simulink model "attitude_control_using_cots_rws_2ucubesat_final"  (R2019b)
settings: Solver=VariableStepAuto  StartTime=0.0  StopTime=5  RelTol=1e-3
libraries: dspmtrx3 x1, sharedutil x1, vrlib x1
settings Model: Creator=Asmaa  LastModifiedBy=AYSHA ALHARAM

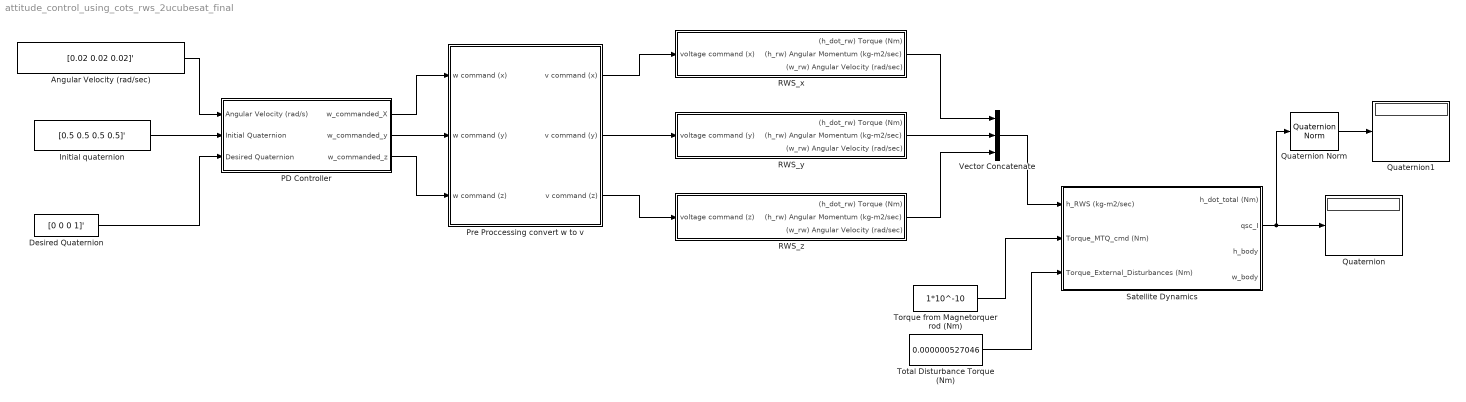
== system attitude_control_using_cots_rws_2ucubesat_final ==
  Angular Velocity (rad/sec) : Constant  Value=[0.02 0.02 0.02]'
  Desired Quaternion : Constant  Value=[0 0 0 1]'
  Initial quaternion : Constant  Value=[0.5 0.5 0.5 0.5]'
  PD Controller : Subsystem
  "Pre Proccessing convert w to v " : Subsystem
  Quaternion : Display
  Quaternion Norm : sharedutil/Quaternion Norm  aMode=aMode
      settings: SourceProductName=Aerospace Blockset  SourceProductBaseCode=AE
  Quaternion1 : Display
  "RWS_x " : Subsystem
  RWS_y : Subsystem
  RWS_z : Subsystem
  Satellite Dynamics : Subsystem
  Torque from Magnetorquer rod (Nm) : Constant  Value=1*10^-10
  Total Disturbance Torque (Nm) : Constant  Value=0.000000527046
  Vector Concatenate : Concatenate  NumInputs=3
  wires:
  "RWS_x "/2((h_rw) Angular Momentum (kg-m2/sec)) -> Vector Concatenate/1
  RWS_y/2((h_rw) Angular Momentum (kg-m2/sec)) -> Vector Concatenate/2
  RWS_z/2((h_rw) Angular Momentum (kg-m2/sec)) -> Vector Concatenate/3
  Vector Concatenate/1 -> Satellite Dynamics/1(h_RWS (kg-m2/sec))
  Total Disturbance Torque (Nm)/1 -> Satellite Dynamics/3(Torque_External_Disturbances (Nm))
  Satellite Dynamics/2(qsc_I) -> Quaternion/1, Quaternion Norm/1
  Initial quaternion/1 -> PD Controller/2(Initial Quaternion)
  PD Controller/1(w_commanded_X) -> "Pre Proccessing convert w to v "/1(w command (x))
  PD Controller/2(w_commanded_y) -> "Pre Proccessing convert w to v "/2(w command (y))
  PD Controller/3(w_commanded_z) -> "Pre Proccessing convert w to v "/3(w command (z))
  "Pre Proccessing convert w to v "/1(v command (x)) -> "RWS_x "/1(voltage command (x))
  "Pre Proccessing convert w to v "/2(v command (y)) -> RWS_y/1(voltage command (y))
  "Pre Proccessing convert w to v "/3(v command (z)) -> RWS_z/1(voltage command (z))
  Desired Quaternion/1 -> PD Controller/3(Desired Quaternion)
  Angular Velocity (rad/sec)/1 -> PD Controller/1(Angular Velocity (rad/s))
  Torque from Magnetorquer rod (Nm)/1 -> Satellite Dynamics/2(Torque_MTQ_cmd (Nm))
  Quaternion Norm/1 -> Quaternion1/1

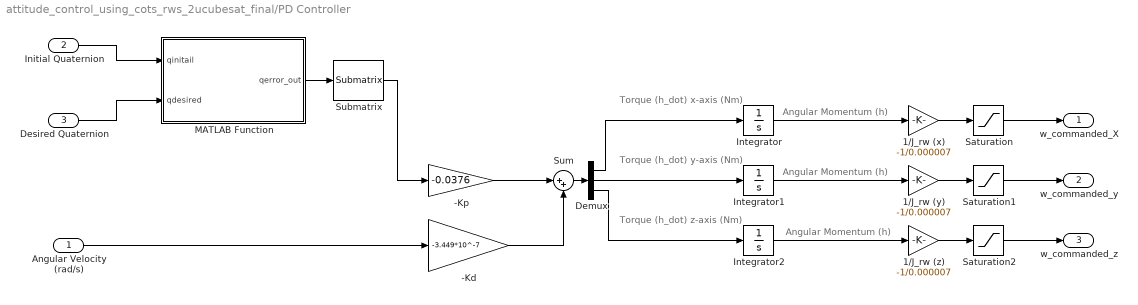
== system attitude_control_using_cots_rws_2ucubesat_final/PD Controller ==
  note: Angular Momentum (h)
  note: Torque (h_dot) x-axis (Nm)
  note: Torque (h_dot) y-axis (Nm)
  note: Torque (h_dot) z-axis (Nm)
  note: Angular Momentum (h)
  note: Angular Momentum (h)
  Angular Velocity (rad/s) : Inport
  Initial Quaternion : Inport  Port=2
  Desired Quaternion : Inport  Port=3
  -Kd : Gain  Gain=-3.449*10^-7
  -Kp : Gain  Gain=-0.0376
  1/J_rw (x) : Gain  Gain=-1/0.000007
  1/J_rw (y) : Gain  Gain=-1/0.000007
  1/J_rw (z) : Gain  Gain=-1/0.000007
  Demux : Demux  Outputs=3
  Integrator : Integrator
  Integrator1 : Integrator
  Integrator2 : Integrator
  MATLAB Function : MATLAB Function  TreatAsAtomicUnit=on
  Saturation : Saturate  UpperLimit=733.038285  LowerLimit=-733.038285  OutMin=-733.038286  OutMax=[733.038286]
  Saturation1 : Saturate  UpperLimit=733.038285  LowerLimit=-733.038285  OutMin=-733.038286  OutMax=[733.038286]
  Saturation2 : Saturate  UpperLimit=733.038285  LowerLimit=-733.038285  OutMin=-733.038286  OutMax=[733.038286]
  Submatrix : dspmtrx3/Submatrix  RowSpan=Range of rows  RowStartMode=Index  RowStartIndex=2  RowEndMode=Last  RowEndIndex=1  ColSpan=Range of columns  ColStartMode=First  ColStartIndex=1  ColEndMode=Last  ColEndIndex=1
  Sum : Sum  Inputs=|++
  w_commanded_X : Outport
  w_commanded_y : Outport  Port=2
  w_commanded_z : Outport  Port=3
  wires:
  Demux/3 -> Integrator2/1
  -Kd/1 -> Sum/2
  -Kp/1 -> Sum/1
  Sum/1 -> Demux/1
  Demux/2 -> Integrator1/1
  Integrator/1 -> 1/J_rw (x)/1
  Integrator1/1 -> 1/J_rw (y)/1
  Integrator2/1 -> 1/J_rw (z)/1
  Demux/1 -> Integrator/1
  1/J_rw (y)/1 -> Saturation1/1
  1/J_rw (z)/1 -> Saturation2/1
  Angular Velocity (rad/s)/1 -> -Kd/1
  1/J_rw (x)/1 -> Saturation/1
  Saturation/1 -> w_commanded_X/1
  Saturation1/1 -> w_commanded_y/1
  Saturation2/1 -> w_commanded_z/1
  Initial Quaternion/1 -> MATLAB Function/1(qinitail)
  Desired Quaternion/1 -> MATLAB Function/2(qdesired)
  MATLAB Function/1(qerror_out) -> Submatrix/1
  Submatrix/1 -> -Kp/1

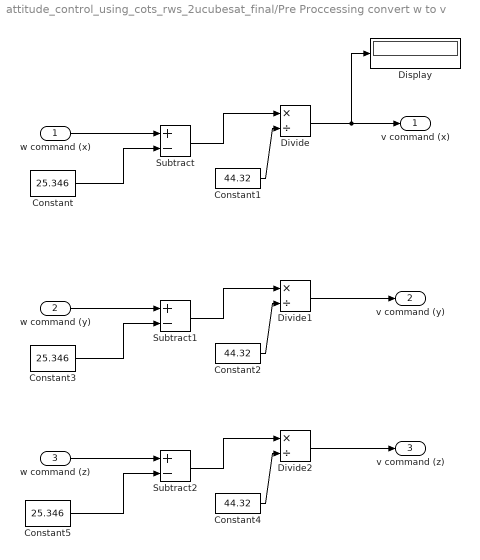
== system attitude_control_using_cots_rws_2ucubesat_final/Pre Proccessing convert w to v  ==
  w command (x) : Inport
  w command (y) : Inport  Port=2
  w command (z) : Inport  Port=3
  Constant : Constant  Value=25.346
  Constant1 : Constant  Value=44.32
  Constant2 : Constant  Value=44.32
  Constant3 : Constant  Value=25.346
  Constant4 : Constant  Value=44.32
  Constant5 : Constant  Value=25.346
  Display : Display
  Divide : Product  Inputs=*/
  Divide1 : Product  Inputs=*/
  Divide2 : Product  Inputs=*/
  Subtract : Sum  Inputs=+-
  Subtract1 : Sum  Inputs=+-
  Subtract2 : Sum  Inputs=+-
  v command (x) : Outport
  v command (y) : Outport  Port=2
  v command (z) : Outport  Port=3
  wires:
  w command (x)/1 -> Subtract/1
  Constant/1 -> Subtract/2
  Subtract/1 -> Divide/1
  Constant1/1 -> Divide/2
  Divide/1 -> Display/1, v command (x)/1
  Subtract1/1 -> Divide1/1
  Constant2/1 -> Divide1/2
  w command (y)/1 -> Subtract1/1
  Divide1/1 -> v command (y)/1
  Constant3/1 -> Subtract1/2
  w command (z)/1 -> Subtract2/1
  Constant4/1 -> Divide2/2
  Divide2/1 -> v command (z)/1
  Constant5/1 -> Subtract2/2
  Subtract2/1 -> Divide2/1

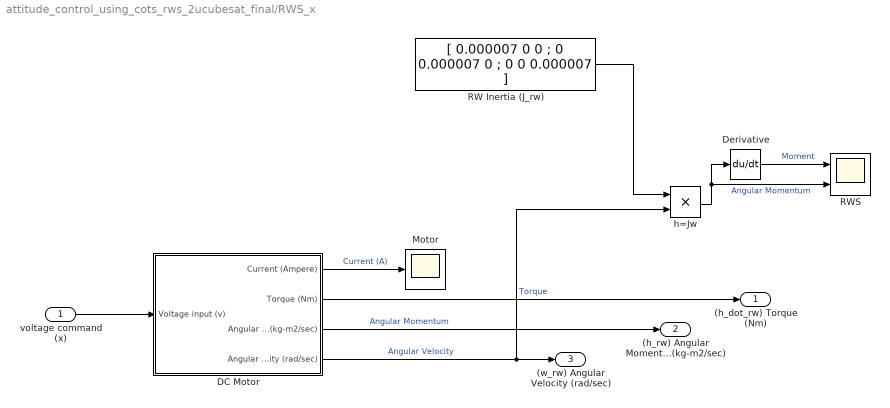
== system attitude_control_using_cots_rws_2ucubesat_final/RWS_x  ==
  voltage command (x) : Inport
  DC Motor : Subsystem
  Derivative : Derivative
  Motor : Scope
  RW Inertia (J_rw) : Constant  Value=[ 0.000007 0 0 ; 0 0.000007 0 ; 0 0 0.000007 ]
  RWS : Scope  NumInputPorts=2
  h=Jw : Product
  (h_dot_rw) Torque (Nm) : Outport
  (h_rw) Angular Momentum (kg-m2/sec) : Outport  Port=2
  (w_rw) Angular Velocity (rad/sec) : Outport  Port=3
  wires:
  RW Inertia (J_rw)/1 -> h=Jw/1
  DC Motor/2(Torque (Nm)) -> (h_dot_rw) Torque (Nm)/1  "Torque"
  h=Jw/1 -> Derivative/1, RWS/2  "Angular Momentum"
  voltage command (x)/1 -> DC Motor/1(Voltage input (v))
  Derivative/1 -> RWS/1  "Moment"
  DC Motor/4(Angular Velocity (rad/sec)) -> (w_rw) Angular Velocity (rad/sec)/1, h=Jw/2  "Angular Velocity"
  DC Motor/1(Current (Ampere)) -> Motor/1  "Current (A)"
  DC Motor/3(Angular Momentum (kg-m2/sec)) -> (h_rw) Angular Momentum (kg-m2/sec)/1  "Angular Momentum"

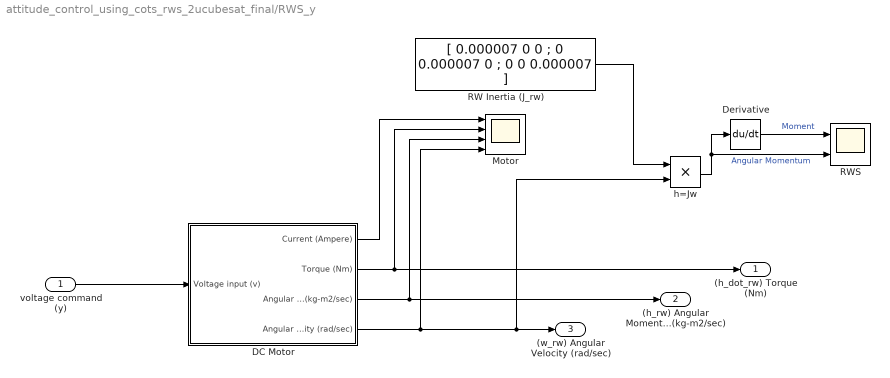
== system attitude_control_using_cots_rws_2ucubesat_final/RWS_y ==
  voltage command (y) : Inport
  DC Motor : Subsystem
  Derivative : Derivative
  Motor : Scope  NumInputPorts=4
  RW Inertia (J_rw) : Constant  Value=[ 0.000007 0 0 ; 0 0.000007 0 ; 0 0 0.000007 ]
  RWS : Scope  NumInputPorts=2
  h=Jw : Product
  (h_dot_rw) Torque (Nm) : Outport
  (h_rw) Angular Momentum (kg-m2/sec) : Outport  Port=2
  (w_rw) Angular Velocity (rad/sec) : Outport  Port=3
  wires:
  DC Motor/2(Torque (Nm)) -> (h_dot_rw) Torque (Nm)/1, Motor/2
  h=Jw/1 -> Derivative/1, RWS/2  "Angular Momentum"
  voltage command (y)/1 -> DC Motor/1(Voltage input (v))
  Derivative/1 -> RWS/1  "Moment"
  DC Motor/4(Angular Velocity (rad/sec)) -> Motor/4, (w_rw) Angular Velocity (rad/sec)/1, h=Jw/2
  DC Motor/1(Current (Ampere)) -> Motor/1
  DC Motor/3(Angular Momentum (kg-m2/sec)) -> (h_rw) Angular Momentum (kg-m2/sec)/1, Motor/3
  RW Inertia (J_rw)/1 -> h=Jw/1

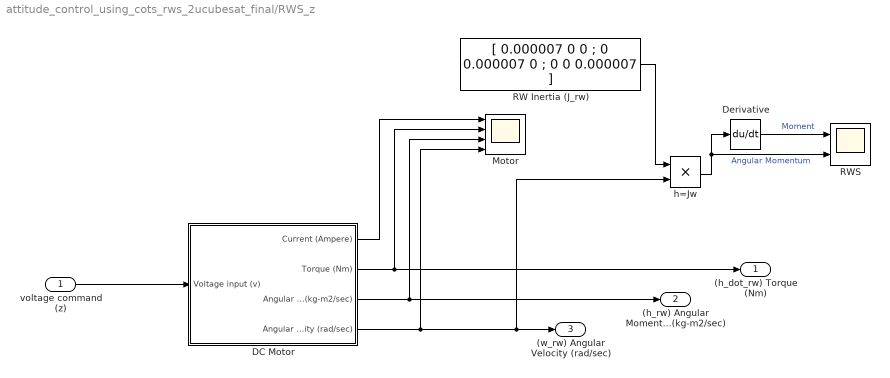
== system attitude_control_using_cots_rws_2ucubesat_final/RWS_z ==
  voltage command (z) : Inport
  DC Motor : Subsystem
  Derivative : Derivative
  Motor : Scope  NumInputPorts=4
  RW Inertia (J_rw) : Constant  Value=[ 0.000007 0 0 ; 0 0.000007 0 ; 0 0 0.000007 ]
  RWS : Scope  NumInputPorts=2
  h=Jw : Product
  (h_dot_rw) Torque (Nm) : Outport
  (h_rw) Angular Momentum (kg-m2/sec) : Outport  Port=2
  (w_rw) Angular Velocity (rad/sec) : Outport  Port=3
  wires:
  DC Motor/2(Torque (Nm)) -> (h_dot_rw) Torque (Nm)/1, Motor/2
  h=Jw/1 -> Derivative/1, RWS/2  "Angular Momentum"
  voltage command (z)/1 -> DC Motor/1(Voltage input (v))
  Derivative/1 -> RWS/1  "Moment"
  DC Motor/4(Angular Velocity (rad/sec)) -> Motor/4, (w_rw) Angular Velocity (rad/sec)/1, h=Jw/2
  DC Motor/1(Current (Ampere)) -> Motor/1
  DC Motor/3(Angular Momentum (kg-m2/sec)) -> (h_rw) Angular Momentum (kg-m2/sec)/1, Motor/3
  RW Inertia (J_rw)/1 -> h=Jw/1

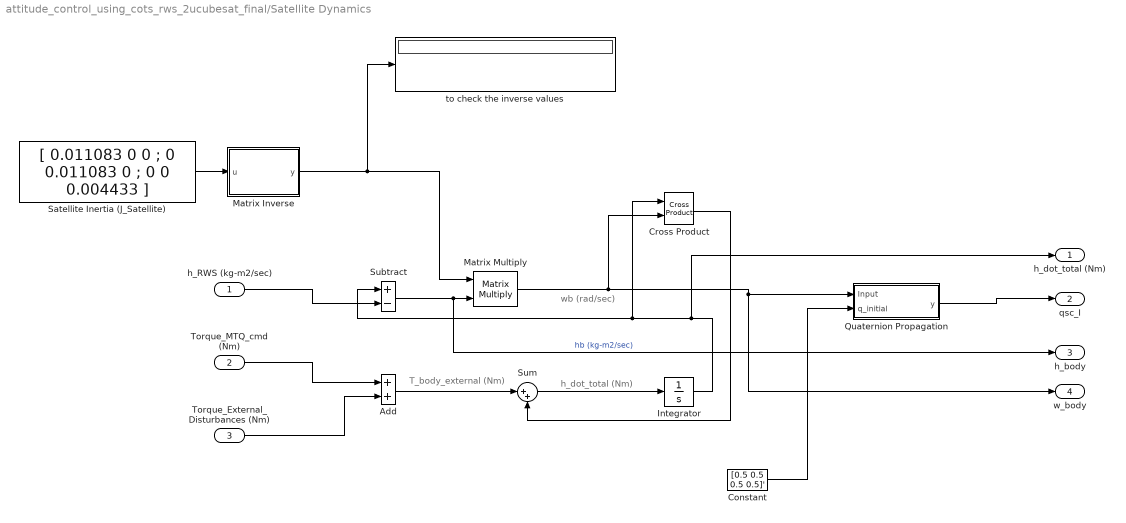
== system attitude_control_using_cots_rws_2ucubesat_final/Satellite Dynamics ==
  note: wb (rad/sec)
  note: T_body_external (Nm)
  note: h_dot_total (Nm)
  h_RWS (kg-m2/sec) : Inport
  Torque_MTQ_cmd (Nm) : Inport  Port=2
  Torque_External_Disturbances (Nm) : Inport  Port=3
  Add : Sum
  Constant : Constant  Value=[0.5 0.5 0.5 0.5]'
  Cross Product : vrlib/Utilities/Cross Product
  Integrator : Integrator
  Matrix Inverse : MATLAB Function  TreatAsAtomicUnit=on
  Matrix Multiply : Product  Multiplication=Matrix(*)
  "Quaternion Propagation " : Subsystem
  Satellite Inertia (J_Satellite) : Constant  Value=[ 0.011083 0 0 ; 0 0.011083 0 ; 0 0 0.004433 ]
  Subtract : Sum  Inputs=+-
  Sum : Sum  Inputs=|++
  to check the inverse values : Display
  h_dot_total (Nm) : Outport
  qsc_I : Outport  Port=2
  h_body : Outport  Port=3
  w_body : Outport  Port=4
  wires:
  Torque_MTQ_cmd (Nm)/1 -> Add/1
  Torque_External_Disturbances (Nm)/1 -> Add/2
  Add/1 -> Sum/1
  Sum/1 -> Integrator/1
  h_RWS (kg-m2/sec)/1 -> Subtract/2
  Subtract/1 -> h_body/1, Matrix Multiply/2  "hb (kg-m2/sec)"
  Matrix Inverse/1(y) -> to check the inverse values/1, Matrix Multiply/1
  Cross Product/1 -> Sum/2
  "Quaternion Propagation "/1(y) -> qsc_I/1
  Satellite Inertia (J_Satellite)/1 -> Matrix Inverse/1(u)
  Matrix Multiply/1 -> Cross Product/2, "Quaternion Propagation "/1(Input), w_body/1
  Integrator/1 -> h_dot_total (Nm)/1, Cross Product/1, Subtract/1
  Constant/1 -> "Quaternion Propagation "/2(q_initial)

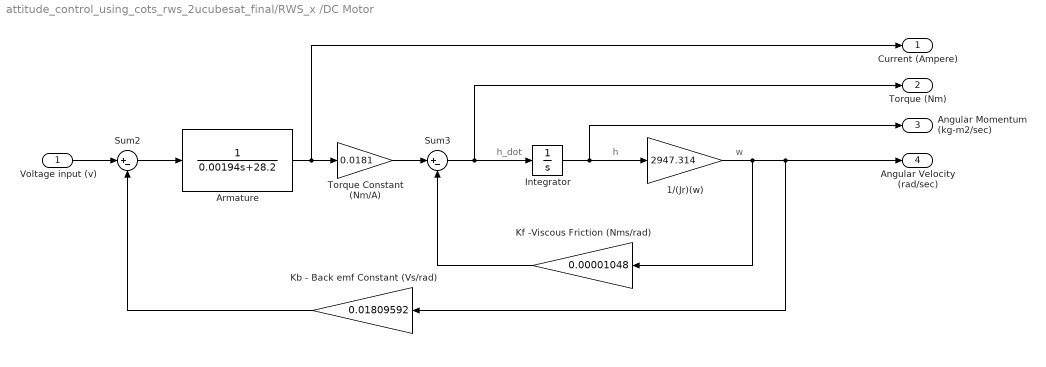
== system attitude_control_using_cots_rws_2ucubesat_final/RWS_x /DC Motor ==
  note: h_dot
  note: h
  note: w
  Voltage input (v) : Inport
  1/(Jr)(w) : Gain  Gain=2947.314
  Armature : TransferFcn  Denominator=[0.00194 28.2]
  Integrator : Integrator
  Kb - Back emf Constant (Vs/rad) : Gain  Gain=0.01809592
  Kf -Viscous Friction (Nms/rad) : Gain  Gain=0.00001048
  Sum2 : Sum  Inputs=|+-
  Sum3 : Sum  Inputs=|+-
  Torque Constant (Nm/A) : Gain  Gain=0.0181
  Current (Ampere) : Outport
  Torque (Nm) : Outport  Port=2
  Angular Momentum (kg-m2/sec) : Outport  Port=3
  Angular Velocity (rad/sec) : Outport  Port=4
  wires:
  Sum3/1 -> Integrator/1, Torque (Nm)/1
  Torque Constant (Nm/A)/1 -> Sum3/1
  Kb - Back emf Constant (Vs/rad)/1 -> Sum2/2
  Kf -Viscous Friction (Nms/rad)/1 -> Sum3/2
  Voltage input (v)/1 -> Sum2/1
  1/(Jr)(w)/1 -> Angular Velocity (rad/sec)/1, Kb - Back emf Constant (Vs/rad)/1, Kf -Viscous Friction (Nms/rad)/1
  Armature/1 -> Current (Ampere)/1, Torque Constant (Nm/A)/1
  Sum2/1 -> Armature/1
  Integrator/1 -> Angular Momentum (kg-m2/sec)/1, 1/(Jr)(w)/1

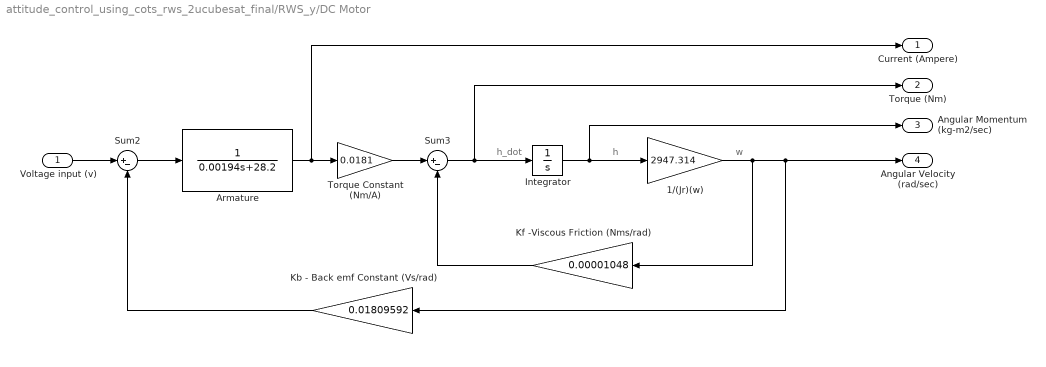
== system attitude_control_using_cots_rws_2ucubesat_final/RWS_y/DC Motor ==
  note: h_dot
  note: h
  note: w
  Voltage input (v) : Inport
  1/(Jr)(w) : Gain  Gain=2947.314
  Armature : TransferFcn  Denominator=[0.00194 28.2]
  Integrator : Integrator
  Kb - Back emf Constant (Vs/rad) : Gain  Gain=0.01809592
  Kf -Viscous Friction (Nms/rad) : Gain  Gain=0.00001048
  Sum2 : Sum  Inputs=|+-
  Sum3 : Sum  Inputs=|+-
  Torque Constant (Nm/A) : Gain  Gain=0.0181
  Current (Ampere) : Outport
  Torque (Nm) : Outport  Port=2
  Angular Momentum (kg-m2/sec) : Outport  Port=3
  Angular Velocity (rad/sec) : Outport  Port=4
  wires:
  Sum3/1 -> Integrator/1, Torque (Nm)/1
  Torque Constant (Nm/A)/1 -> Sum3/1
  Kb - Back emf Constant (Vs/rad)/1 -> Sum2/2
  Kf -Viscous Friction (Nms/rad)/1 -> Sum3/2
  Voltage input (v)/1 -> Sum2/1
  1/(Jr)(w)/1 -> Angular Velocity (rad/sec)/1, Kb - Back emf Constant (Vs/rad)/1, Kf -Viscous Friction (Nms/rad)/1
  Armature/1 -> Current (Ampere)/1, Torque Constant (Nm/A)/1
  Sum2/1 -> Armature/1
  Integrator/1 -> Angular Momentum (kg-m2/sec)/1, 1/(Jr)(w)/1

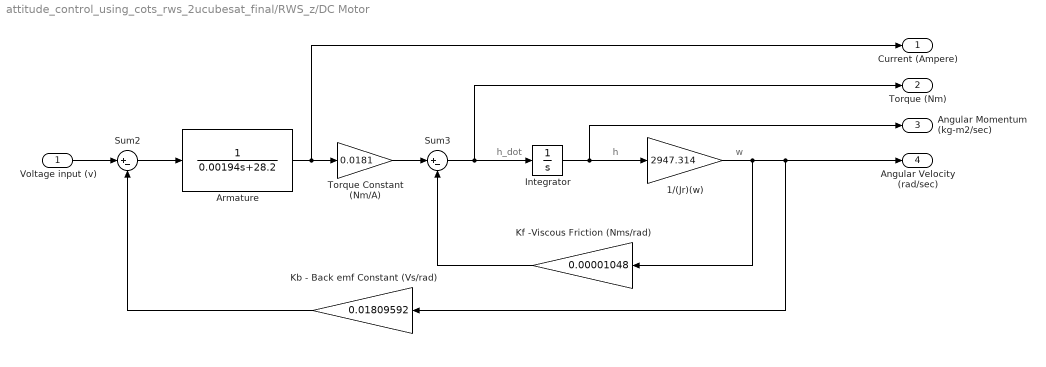
== system attitude_control_using_cots_rws_2ucubesat_final/RWS_z/DC Motor ==
  note: h_dot
  note: h
  note: w
  Voltage input (v) : Inport
  1/(Jr)(w) : Gain  Gain=2947.314
  Armature : TransferFcn  Denominator=[0.00194 28.2]
  Integrator : Integrator
  Kb - Back emf Constant (Vs/rad) : Gain  Gain=0.01809592
  Kf -Viscous Friction (Nms/rad) : Gain  Gain=0.00001048
  Sum2 : Sum  Inputs=|+-
  Sum3 : Sum  Inputs=|+-
  Torque Constant (Nm/A) : Gain  Gain=0.0181
  Current (Ampere) : Outport
  Torque (Nm) : Outport  Port=2
  Angular Momentum (kg-m2/sec) : Outport  Port=3
  Angular Velocity (rad/sec) : Outport  Port=4
  wires:
  Sum3/1 -> Integrator/1, Torque (Nm)/1
  Torque Constant (Nm/A)/1 -> Sum3/1
  Kb - Back emf Constant (Vs/rad)/1 -> Sum2/2
  Kf -Viscous Friction (Nms/rad)/1 -> Sum3/2
  Voltage input (v)/1 -> Sum2/1
  1/(Jr)(w)/1 -> Angular Velocity (rad/sec)/1, Kb - Back emf Constant (Vs/rad)/1, Kf -Viscous Friction (Nms/rad)/1
  Armature/1 -> Current (Ampere)/1, Torque Constant (Nm/A)/1
  Sum2/1 -> Armature/1
  Integrator/1 -> Angular Momentum (kg-m2/sec)/1, 1/(Jr)(w)/1

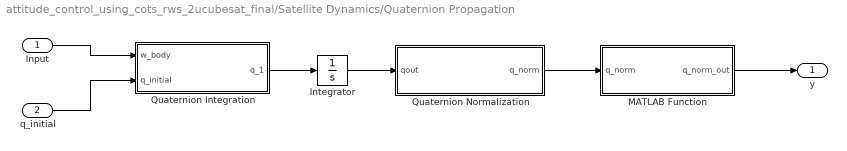
== system attitude_control_using_cots_rws_2ucubesat_final/Satellite Dynamics/Quaternion Propagation  ==
  Input : Inport
  q_initial : Inport  Port=2
  Integrator : Integrator
  MATLAB Function : MATLAB Function  TreatAsAtomicUnit=on
  Quaternion Integration : MATLAB Function  TreatAsAtomicUnit=on
  Quaternion Normalization : MATLAB Function  TreatAsAtomicUnit=on
  y : Outport
  wires:
  Integrator/1 -> Quaternion Normalization/1(qout)
  Quaternion Integration/1(q_1) -> Integrator/1
  q_initial/1 -> Quaternion Integration/2(q_initial)
  Input/1 -> Quaternion Integration/1(w_body)
  Quaternion Normalization/1(q_norm) -> MATLAB Function/1(q_norm)
  MATLAB Function/1(q_norm_out) -> y/1

== matlab function attitude_control_using_cots_rws_2ucubesat_final/Satellite Dynamics/Quaternion Propagation /Quaternion Integration ==
  data: w_body input; q_1 output; q_initial input
function q_1 = Qderivative(w_body,q_initial)
    q_last = q_initial(1);  
    q = q_initial(2:4); 
    M = [0,-q(3),q(2);q(3),0,-q(1);-q(2),q(1),0];   
    q_1 = 0.5*[q_last*eye(3)+M; -q']*w_body;
end

== matlab function attitude_control_using_cots_rws_2ucubesat_final/Satellite Dynamics/Matrix Inverse ==
  data: u input; y output
function y = fcn(u)

y = inv(u);

== matlab function attitude_control_using_cots_rws_2ucubesat_final/Satellite Dynamics/Quaternion Propagation /Quaternion Normalization ==
  data: qout input; q_norm output
 function q_norm= Q_norm(qout) 
 q_norm = zeros(4,1);   
 qtemp = qout(1)*qout(1) + qout(2)*qout(2) + qout(3)*qout(3) + qout(4)*qout(4);   
 if qtemp <= 1.0e-10      
     for i=1:3         
         q_norm(i) = 0;   
     end
     q_norm(1) = 1.0;   
 else
     qtemp = sqrt(qtemp);   
     for i=1:4       
         q_norm(i) = qout(i)/qtemp;  
     end
     
 end

== matlab function attitude_control_using_cots_rws_2ucubesat_final/Satellite Dynamics/Quaternion Propagation /MATLAB Function ==
  data: q_norm input; q_norm_out output
function q_norm_out = flipsign(q_norm)

 if q_norm(1) < 0.0 
     q_norm_out = -q_norm;
 else
     q_norm_out= q_norm;
 end

== matlab function attitude_control_using_cots_rws_2ucubesat_final/PD Controller/MATLAB Function ==
  data: qinitail input; qerror_out output; qdesired input
  function qerror_out= Qua_err(qinitail, qdesired)
  qdesired = qdesired(:);
  qest = qinitail(2:4);
  qlast = qinitail(1);
  M = [0,-qest(3),qest(2);
      qest(3),0,-qest(1);
      -qest(2),qest(1),0];
  Qerr = [qlast*eye(3)-M,-qest;qest',qlast];
  qerror = Qerr*qdesired;
  
  if qerror(1) < 0.0 
     qerror_out = -qerror;
  else
      qerror_out= qerror;
  end
  end
